simulink model "quadruple_simulink_block"  (R2021b)
settings: Solver=FixedStepAuto  StartTime=0.0  StopTime=inf  FixedStep=0.5  RelTol=1e-3
undefined symbols (not defined in the file or in its folder): cte
libraries: sldrtlib x1
settings Model: Creator=IST  LastModifiedBy=IST

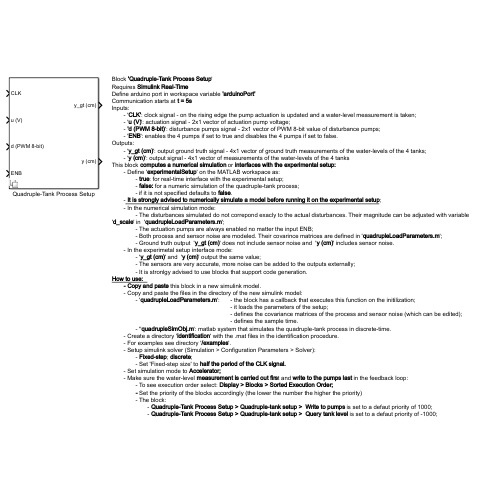
[thumbnail: Simulink's stored preview of the top-level diagram]
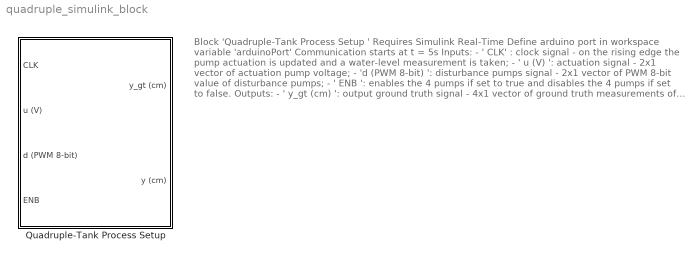
== system quadruple_simulink_block ==
  note: Block 'Quadruple-Tank Process Setup '
      | Requires Simulink Real-Time
      | Define arduino port in workspace variable 'arduinoPort'
      | Communication starts at t = 5s
      | Inputs:
      | - ' CLK' : clock signal - on the rising edge the pump actuation is updated and a water-level measurement is taken;
      | - ' u (V) ': actuation signal - 2x1 vector of actuation pump voltage;
      | - 'd (PWM 8-bit) ': disturbance pumps signal - 2x1 vector of PWM 8-bit value of disturbance pumps;
      | - ' ENB ': enables the 4 pumps if set to true and disables the 4 pumps if set to false.
      | Outputs:
      | - ' y_gt (cm) ': output ground truth signal - 4x1 vector of ground truth measurements of the water-levels of the 4 tanks;
      | - ' y (cm) ': output signal - 4x1 vector of measurements of the water-levels of the 4 tanks
      | This block computes a numerical simulation or interfaces with the experimental setup:
      | - Define ' experimentalSetup ' on the MATLAB workspace as:
      | - true : for real-time interface with the experimental setup;
      | - false: for a numeric simulation of the quadruple-tank process;
      | - if it is not specified defaults to false .
      | - It is strongly advised to numerically simulate a model before running it on the experimental setup ;
      | - In the numerical simulation mode:
      | - The disturbances simulated do not correpond exacly to the actual disturbances. Their magnitude can be adjusted with variable ' d_scale ' in ' quadrupleLoadParameters.m ';
      | - The actuation pumps are always enabled no matter the input ENB;
      | - Both process and sensor noise are modeled. Their covarince matrices are defined in ' quadrupleLoadParameters.m ';
      | - Ground truth output ' y_gt (cm) ' does not include sensor noise and ' y (cm) ' includes sensor noise.
      | - In the experimetal setup interface mode:
      | - ' y_gt (cm) ' and ' y (cm) ' output the same value;
      | - The sensors are very accurate, more noise can be added to the outputs externally;
      | - It is stronlgy advised to use blocks that support code generation.
      | How to use:
      | - Copy and paste this block in a new simulink model.
      | - Copy and paste the files in the directory of the new simulink model:
      | - ' quadrupleLoadParameters.m ': - the block has a callback that executes this function on the initilization;
      | - it loads the parameters of the setup;
      | - defines the covariance matrices of the process and sensor noise (which can be edited);
      | - defines the sample time.
      | - '' quadrupleSimObj.m ': matlab system that simulates the quadruple-tank process in discrete-time.
      | - Create a directory ' identification ' with the .mat files in the identification procedure.
      | - For examples see directory ' /examples '.
      | - Setup simulink solver (Simulation > Configuration Parameters > Solver):
      | - Fixed-step ; discrete ;
      | - Set 'Fixed-step size' to half the period of the CLK signal.
      | - Set simulation mode to Accelerator;
      | - Make sure the water-level measurement is carried out firs t and write to the pumps last in the feedback loop:
      | - To see execution order select: Display > Blocks > Sorted Execution Order;
      | - Set the priority of the blocks accordingly (the lower the number the higher the priority)
      | - The block:
      | - Quadruple-Tank Process Setup > Quadruple-tank setup > Write to pumps is set to a defaut priority of 1000;
      | - Quadruple-Tank Process Setup > Quadruple-tank setup > Query tank level is set to a defaut priority of -1000;
  Quadruple-Tank Process Setup : Subsystem  InitFcn=|  StopFcn=|  Variant=on
      InitFcn=|
      | % Load parameters
      | cte = quadrupleLoadParameters();
      | % Select simulation mode if unspecified
      | if ~exist('experimentalSetup')
      | experimentalSetup = false;
      | end
      | if experimentalSetup
      | if exist('arduinoPort')
      | if ~isempty(instrfind)
      | fclose(instrfind);
      | delete(instrfind);
      | end
      | arduino = serial(arduinoPort,...
      |                 'BaudRate',9600,...
      |                 'ByteOrder','bigEndian',...
      |                 'DataBits',8,...
      |                 'StopBits',1,...
      |                 'Terminator','');
      | arduino.Parity = 'none';
      | fopen(arduino);
      | else
      | error("Error: Arduino port undefined. Define the port in workspace variable 'arduinoPort'.");
      | end
      | end
      StopFcn=|
      | if experimentalSetup
      | fclose(arduino);
      | end

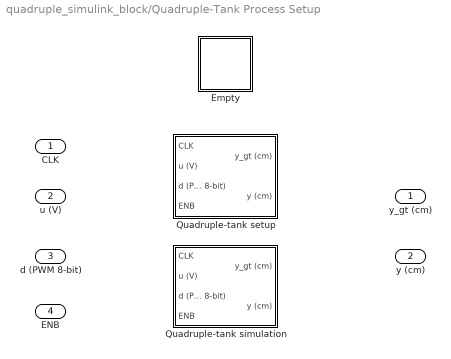
== system quadruple_simulink_block/Quadruple-Tank Process Setup ==
  CLK : Inport
  u (V) : Inport  Port=2
  d (PWM 8-bit) : Inport  Port=3
  ENB : Inport  Port=4
  Empty : Subsystem  VariantControl=%
  Quadruple-tank setup : Subsystem  VariantControl=experimentalSetup == true
  Quadruple-tank simulation : Subsystem  Priority=4  VariantControl=experimentalSetup == false
  y_gt (cm) : Outport  VectorParamsAs1DForOutWhenUnconnected=off
  y (cm) : Outport  Port=2  VectorParamsAs1DForOutWhenUnconnected=off

== system quadruple_simulink_block/Quadruple-Tank Process Setup/Empty ==

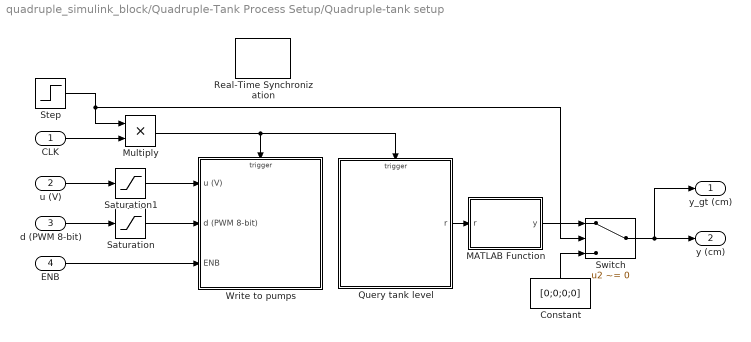
== system quadruple_simulink_block/Quadruple-Tank Process Setup/Quadruple-tank setup ==
  CLK : Inport
  u (V) : Inport  Port=2
  d (PWM 8-bit) : Inport  Port=3
  ENB : Inport  Port=4
  Constant : Constant  Value=[0;0;0;0]
  MATLAB Function : MATLAB Function  TreatAsAtomicUnit=on
  Multiply : Product
  Query tank level : Subsystem  Priority=1
  Real-Time Synchronization : sldrtlib/Real-Time Synchronization  Priority=5  SampleTime=0.5  MaxMissedTicks=10  ShowMissedTicks=off  YieldWhenWaiting=off
  Saturation : Saturate  UpperLimit=255  LowerLimit=0
  Saturation1 : Saturate  UpperLimit=cte.uMax  LowerLimit=cte.uMin
  Step : Step  Time=5  SampleTime=0
  Switch : Switch  Criteria=u2 ~= 0
  Write to pumps : Subsystem  Priority=100
  y_gt (cm) : Outport  VectorParamsAs1DForOutWhenUnconnected=off
  y (cm) : Outport  Port=2  VectorParamsAs1DForOutWhenUnconnected=off
  wires:
  ENB/1 -> Write to pumps/3(ENB)
  Query tank level/1(r) -> MATLAB Function/1(r)
  d (PWM 8-bit)/1 -> Saturation/1
  Saturation/1 -> Write to pumps/2(d (PWM 8-bit))
  u (V)/1 -> Saturation1/1
  Saturation1/1 -> Write to pumps/1(u (V))
  MATLAB Function/1(y) -> Switch/1
  Switch/1 -> y_gt (cm)/1, y (cm)/1
  Constant/1 -> Switch/3
  Step/1 -> Multiply/1, Switch/2
  CLK/1 -> Multiply/2
  Multiply/1 -> Write to pumps/Trigger, Query tank level/Trigger

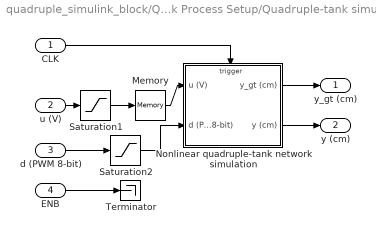
== system quadruple_simulink_block/Quadruple-Tank Process Setup/Quadruple-tank simulation ==
  CLK : Inport
  u (V) : Inport  Port=2
  d (PWM 8-bit) : Inport  Port=3
  ENB : Inport  Port=4
  Memory : Memory
  Nonlinear quadruple-tank network simulation : Subsystem  Priority=10
  Saturation1 : Saturate  UpperLimit=cte.uMax  LowerLimit=cte.uMin
  Saturation2 : Saturate  UpperLimit=2^8-1  LowerLimit=0
  Terminator : Terminator
  y_gt (cm) : Outport  VectorParamsAs1DForOutWhenUnconnected=off
  y (cm) : Outport  Port=2  VectorParamsAs1DForOutWhenUnconnected=off
  wires:
  CLK/1 -> Nonlinear quadruple-tank network simulation/Trigger
  Nonlinear quadruple-tank network simulation/2(y (cm)) -> y (cm)/1
  ENB/1 -> Terminator/1
  Memory/1 -> Nonlinear quadruple-tank network simulation/1(u (V))
  Nonlinear quadruple-tank network simulation/1(y_gt (cm)) -> y_gt (cm)/1
  d (PWM 8-bit)/1 -> Saturation2/1
  u (V)/1 -> Saturation1/1
  Saturation1/1 -> Memory/1
  Saturation2/1 -> Nonlinear quadruple-tank network simulation/2(d (PWM 8-bit))

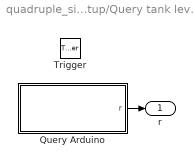
== system quadruple_simulink_block/Quadruple-Tank Process Setup/Quadruple-tank setup/Query tank level ==
  Trigger : TriggerPort  VariantControl=Variant  PortDimensions=1
  Query Arduino : MATLAB Function  TreatAsAtomicUnit=on
  r : Outport  VectorParamsAs1DForOutWhenUnconnected=off
  wires:
  Query Arduino/1(r) -> r/1

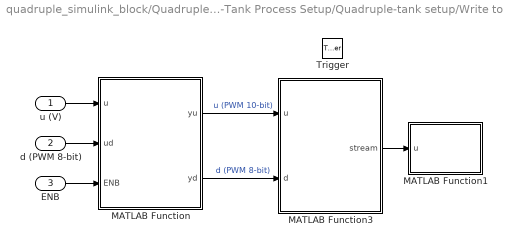
== system quadruple_simulink_block/Quadruple-Tank Process Setup/Quadruple-tank setup/Write to pumps ==
  u (V) : Inport
  d (PWM 8-bit) : Inport  Port=2
  ENB : Inport  Port=3
  Trigger : TriggerPort  VariantControl=Variant  PortDimensions=1
  MATLAB Function : MATLAB Function  TreatAsAtomicUnit=on
  MATLAB Function1 : MATLAB Function  TreatAsAtomicUnit=on
  MATLAB Function3 : MATLAB Function  TreatAsAtomicUnit=on
  wires:
  MATLAB Function/1(yu) -> MATLAB Function3/1(u)  "u (PWM 10-bit)"
  MATLAB Function/2(yd) -> MATLAB Function3/2(d)  "d (PWM 8-bit)"
  u (V)/1 -> MATLAB Function/1(u)
  d (PWM 8-bit)/1 -> MATLAB Function/2(ud)
  ENB/1 -> MATLAB Function/3(ENB)
  MATLAB Function3/1(stream) -> MATLAB Function1/1(u)

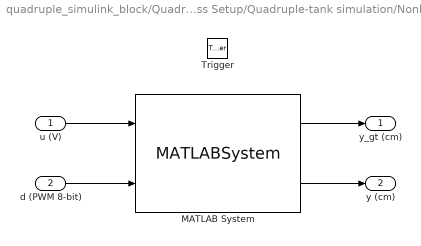
== system quadruple_simulink_block/Quadruple-Tank Process Setup/Quadruple-tank simulation/Nonlinear quadruple-tank network simulation ==
  u (V) : Inport
  d (PWM 8-bit) : Inport  Port=2
  Trigger : TriggerPort  VariantControl=Variant  PortDimensions=1
  MATLAB System : MATLABSystem  System=quadrupleSimObj  SimulateUsing=Interpreted execution
      mask Type: quadrupleSimObj
      mask Display:
      | disp('quadrupleSimObj');
      | port_label('input',1,'u');
      | port_label('input',2,'d');
      | port_label('output',1,'y_gt');
      | port_label('output',2,'y');
  y_gt (cm) : Outport  VectorParamsAs1DForOutWhenUnconnected=off
  y (cm) : Outport  Port=2  VectorParamsAs1DForOutWhenUnconnected=off
  wires:
  u (V)/1 -> MATLAB System/1
  MATLAB System/1 -> y_gt (cm)/1
  MATLAB System/2 -> y (cm)/1
  d (PWM 8-bit)/1 -> MATLAB System/2

== matlab function quadruple_simulink_block/Quadruple-Tank Process Setup/Quadruple-tank setup/Write to pumps/MATLAB Function1 ==
  data: u input
function toArduino(u)
% Find arduino serial object
coder.extrinsic('instrfind'); 
persistent arduino;
if isempty(arduino)
    arduino = instrfind('Status','open','Baud',9600);
end
% Send metadata
fprintf(arduino, "#16");
% Send actuation inputs
fwrite(arduino,u,'uint16');
end

== matlab function quadruple_simulink_block/Quadruple-Tank Process Setup/Quadruple-tank setup/Query tank level/Query Arduino ==
  data: r output
function r = queryArduino()
% Find arduino serial object
coder.extrinsic('instrfind'); 
persistent arduino;
if isempty(arduino)
    arduino = instrfind('Status','open','Baud',9600);
end

% Query arduino
fprintf(arduino, '$');
% Ignore metadata
fread(arduino,[4 1],'uint8');
% Read water-level data
aux = fread(arduino,[5 1],'uint16');
u = zeros(5,1);
u(5) = double(aux(5,1));
for i = 1:4
    u(i) = double(aux(i,1));
    u(i) = (u(5)-u(i))/u(i);
end
r = u(1:4);
end

== matlab function quadruple_simulink_block/Quadruple-Tank Process Setup/Quadruple-tank setup/Write to pumps/MATLAB Function ==
  data: u input; ud input; ENB input; yu output; cte parameter; yd output
function [yu,yd] = pwm_u(u,ud,ENB,cte)
% In u in volts
if ENB
    for i = 1:2
        u(i) = 1023*(cte.c(1,i)*cte.c(3,i)-cte.c(2,i)*cte.k(i)*u(i))/(cte.c(1,i)-cte.k(i)*u(i));
    end
    yu = u;
    yd = ud;
else
    yu = zeros(2,1);
    yd = zeros(2,1);
end

== matlab function quadruple_simulink_block/Quadruple-Tank Process Setup/Quadruple-tank setup/MATLAB Function ==
  data: r input; y output; cte parameter
function y = water_level(r,cte)
y = zeros(4,1);
for i = 1:4
   y(i) = r(i)*cte.dh_dr(i)+cte.h0(i);
end

== matlab function quadruple_simulink_block/Quadruple-Tank Process Setup/Quadruple-tank setup/Write to pumps/MATLAB Function3 ==
  data: u input; stream output; d input
function stream = packPWM10bit(u,d)
    %% Saturation 
    u(u<0) = 0;
    u(u>2^10-1) =2^10-1;
    d(d<0) = 0;
    d(d>2^8-1) =2^8-1;
    %% Pack PWM 
    stream = uint16(zeros(3,1));
    % First two actuation pump signals of 10 bits are sent individually
    stream(1:2) = uint16(round(u)); 
    % Two disturbance pump signals of 8 bits are sent together as a 16 bit
    % uint16_t
    stream(3) = uint16(round(d(1))*2^8+round(d(2)));
end
